simulink model "example_of_relational_operator"  (R2021a)
settings: Solver=VariableStepAuto  StartTime=0.0  StopTime=10.0  MaxStep=1e-3  RelTol=1e-3
libraries: simulink x3
settings Model: Creator=YasserNet  LastModifiedBy=YasserNet

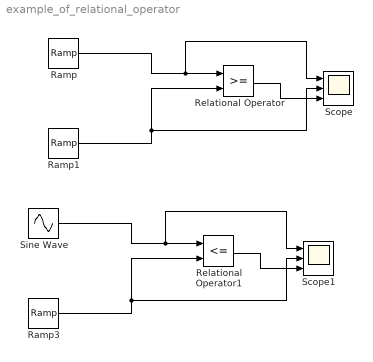
== system example_of_relational_operator ==
  Ramp : simulink/Sources/Ramp  slope=1  start=1  InitialOutput=-4
  Ramp1 : simulink/Sources/Ramp  slope=-1  start=2  InitialOutput=8
  Ramp3 : simulink/Sources/Ramp  slope=-1  start=2  InitialOutput=8
  Relational Operator : RelationalOperator  OutDataTypeStr=boolean  RndMeth=Simplest
  Relational Operator1 : RelationalOperator  Operator=<=  OutDataTypeStr=boolean  RndMeth=Simplest
  Scope : Scope  NumInputPorts=3
  Scope1 : Scope  NumInputPorts=3
  Sine Wave : Sin  Amplitude=4  Frequency=2*2*pi  SampleTime=0
  wires:
  Relational Operator/1 -> Scope/3
  Ramp/1 -> Scope/1, Relational Operator/1
  Ramp1/1 -> Scope/2, Relational Operator/2
  Ramp3/1 -> Relational Operator1/2, Scope1/2
  Sine Wave/1 -> Relational Operator1/1, Scope1/1
  Relational Operator1/1 -> Scope1/3
